simulink model "main_sim"  (Simulink 7.2)
settings: Solver=ode2  SolverMode=SingleTasking  StartTime=0.0  StopTime=tsim_max  FixedStep=dtsim  RelTol=1e-3
StopFcn:
  | %mkplt
undefined symbols (not defined in the file): aero_surf_qbar_off, aero_surf_qbar_on, assertion_time, att_type, att_type_numbers, bb_ellipsoid, bb_params, compute_all_rate_cols, compute_all_vel_cols, constants, cosA, DiscIntNeverNeededParam, dtsim, E_rwy, eow_boundary, full_surf_llim, full_surf_ulim, gain_set, gain_var_struct, MACH, MACH_att_fb, MACH_gain_mat, MACH_mass_IC, MACH_pos_IC, MACH_pqr_Bmat_IC, MACH_pqr_IC, MACH_pqr_u_IC, MACH_quat_IC, MACH_throttle_IC, MACH_U_nom_IC, MACH_vel_Bmat_IC, MACH_vel_cvdnom_IC, MACH_vel_IC, MACH_vel_uold_IC, max_LOS_rate, modes, N_rwy, pos, rcs_cvddes_thresh, reset_camcmd_on_entry, sinA, target_pos_IC, target_range_blind, target_range_detect, target_range_homing, target_vel_IC, trac_params, u_llim, u_ulim, use_auto_att_type, use_eow_as_iv, use_nav, use_pos_fltpath_lim, use_throt_estimate, use_variable_mass, use_wind_est, vel, vel_cmd_ramp_time, x_trac_IC
libraries: simulink x32, mach_lib x26, utility_lib x24, model_lib x15, simulink_need_slupdate x8, models x6
(part 3 of 5)

== system main_sim/claw_main/vel_loops/config_di ==
  cvd_nom : Inport  OutDataType=sfix(16)  OutScaling=2^0
  Bmat : Inport  Port=2  OutDataType=sfix(16)  OutScaling=2^0
  d_old : Inport  Port=3  OutDataType=sfix(16)  OutScaling=2^0
  d_nom : Inport  Port=4  OutDataType=sfix(16)  OutScaling=2^0
  cvd_des : Inport  Port=5  OutDataType=sfix(16)  OutScaling=2^0
  params : Inport  Port=6  OutDataType=sfix(16)  OutScaling=2^0
  di_smn : mach_lib/di_smn  SystemSampleTime=-1
  d_cmd : Outport  OutDataType=sfix(16)  OutScaling=2^0
  cvd_extra : Outport  Port=2  OutDataType=sfix(16)  OutScaling=2^0
  lambda : Outport  Port=3  OutDataType=sfix(16)  OutScaling=2^0
  solve_dat : Outport  Port=4  OutDataType=sfix(16)  OutScaling=2^0
  wires:
  cvd_nom/1 -> di_smn/1
  Bmat/1 -> di_smn/2
  d_old/1 -> di_smn/3
  d_nom/1 -> di_smn/4
  cvd_des/1 -> di_smn/5
  params/1 -> di_smn/6
  di_smn/1 -> d_cmd/1
  di_smn/2 -> cvd_extra/1
  di_smn/3 -> lambda/1
  di_smn/4 -> solve_dat/1

== system main_sim/claw_main/vel_loops/convert accel_cmd to NED_dd_cmd ==
  accel_cmd : Inport  OutDataType=sfix(16)  OutScaling=2^0
  accel_cmd_sw : Inport  Port=2  OutDataType=sfix(16)  OutScaling=2^0
  NEh_d : Inport  Port=3  OutDataType=sfix(16)  OutScaling=2^0
  Merge : Merge  InitialOutput=zeros(3,1)
  MinMax : MinMax  Function=max  OutDataType=sfix(16)  OutScaling=2^0
  NED_dd cmd : Subsystem  TreatAsAtomicUnit=on
  Switch Case : SwitchCase  CaseConditions={1,2}  CaseShowDefault=off
  vchigam_dot cmd : Subsystem  TreatAsAtomicUnit=on
  NEh_dd_cmd : Outport  OutDataType=sfix(16)  OutScaling=2^0
  wires:
  accel_cmd_sw/1 -> MinMax/1
  MinMax/1 -> Switch Case/1
  NEh_d/1 -> vchigam_dot cmd/2(NEh_d)
  vchigam_dot cmd/1(NEh_dd_cmd) -> Merge/2
  Merge/1 -> NEh_dd_cmd/1
  Switch Case/1 -> NED_dd cmd/Action
  Switch Case/2 -> vchigam_dot cmd/Action
  accel_cmd/1 -> vchigam_dot cmd/1(vchigam_dot_cmd), NED_dd cmd/1(NEH_dd_cmd_in)
  NED_dd cmd/1(NEh_dd_cmd) -> Merge/1

== system main_sim/claw_main/vel_loops/from inner ==
  att,T : Inport  OutDataType=sfix(16)  OutScaling=2^0
  Demux1 : Demux  Outputs=[ 2 1 MACH.num_u_throt ]
  Mux1 : Mux  Inputs=2
  Terminator : Terminator
  d_cmd : Outport  OutDataType=sfix(16)  OutScaling=2^0
  wires:
  att,T/1 -> Demux1/1
  Demux1/1 -> Mux1/1
  Mux1/1 -> d_cmd/1
  Demux1/3 -> Mux1/2
  Demux1/2 -> Terminator/1

== system main_sim/claw_main/vel_loops/from quat ==
  e,T : Inport  OutDataType=sfix(16)  OutScaling=2^0
  Demux1 : Demux  Outputs=[ 4 MACH.num_u_throt ]
  Mux1 : Mux  Inputs=2
  Selector1 : Selector  InputPortWidth=3  IndexOptions=Index vector (dialog)  Indices=1:2  OutputSizes=1
  e2att : utility_lib/e2att  SystemSampleTime=-1
  d_cmd : Outport  OutDataType=sfix(16)  OutScaling=2^0
  wires:
  e2att/1 -> Selector1/1
  Selector1/1 -> Mux1/1
  Demux1/2 -> Mux1/2
  Mux1/1 -> d_cmd/1
  Demux1/1 -> e2att/1
  e,T/1 -> Demux1/1

== system main_sim/claw_main/vel_loops/select vel cmd ==
  NEh_dot_current : Inport  OutDataType=sfix(16)  OutScaling=2^0
  cam_current : Inport  Port=2  OutDataType=sfix(16)  OutScaling=2^0
  outer cmd : Inport  Port=3  OutDataType=sfix(16)  OutScaling=2^0
  signal_bus : Inport  Port=4  OutDataType=sfix(16)  OutScaling=2^0
  Bus Selector : BusSelector  OutputSignals=cmd_bus.select_cmd.vel,cmd_bus.autopilot_cmd
  Demux3 : Demux  Outputs=[ MACH.vel_num_cv 1 ]
  Multiport Switch : MultiPortSwitch  zeroidx=on  SaturateOnIntegerOverflow=on
  Mux : Mux  Inputs=2
  Selector1 : Selector  InputPortWidth=4  IndexOptions=Index vector (dialog)  Indices=[1 2 4 3]  OutputSizes=1
  Selector2 : Selector  InputPortWidth=4  IndexOptions=Index vector (dialog)  Indices=[1 2 4 3]  OutputSizes=1
  NEh_dot_cmd : Outport  OutDataType=sfix(16)  OutScaling=2^0
  cam_cmd : Outport  Port=2  OutDataType=sfix(16)  OutScaling=2^0
  cmd : Outport  Port=3  OutDataType=sfix(16)  OutScaling=2^0
  wires:
  Multiport Switch/1 -> cmd/1, Selector2/1
  outer cmd/1 -> Multiport Switch/4
  Bus Selector/1 -> Multiport Switch/1  "<vel>"
  Selector2/1 -> Demux3/1
  Demux3/1 -> NEh_dot_cmd/1
  Demux3/2 -> cam_cmd/1
  Mux/1 -> Selector1/1
  NEh_dot_current/1 -> Mux/1
  Selector1/1 -> Multiport Switch/2
  signal_bus/1 -> Bus Selector/1
  Bus Selector/2 -> Multiport Switch/3  "<autopilot_cmd>"
  cam_current/1 -> Mux/2

== system main_sim/claw_main/vel_loops/set di params ==
  note: Note: dc_fltpath is now computed from NEh_dot.
      | Switch to recover old computation base on NEh_dot_cmd
  NEh_dot_cmd : Inport  OutDataType=sfix(16)  OutScaling=2^0
  full_surf : Inport  Port=2  OutDataType=sfix(16)  OutScaling=2^0
  u_old : Inport  Port=3  OutDataType=sfix(16)  OutScaling=2^0
  uvw : Inport  Port=4  OutDataType=sfix(16)  OutScaling=2^0
  dc_fltpath : Inport  Port=5  OutDataType=sfix(16)  OutScaling=2^0
  Bus Creator1 : BusCreator  Inputs=7
  Bus Selector : BusSelector  OutputSignals=u_ulim,u_llim,u_urlim,u_lrlim
  Bus Selector1 : BusSelector  OutputSignals=throt_ulim,throt_llim
  Constant1 : Constant  Value=MACH.vel_wght_cv  OutDataType=sfix(16)  OutScaling=2^0
  Constant3 : Constant  Value=MACH.vel_u_pref  OutDataType=sfix(16)  OutScaling=2^0
  Constant4 : Constant  Value=MACH.vel_wght_u_pref  OutDataType=sfix(16)  OutScaling=2^0
  Demux1 : Demux  Outputs=[ 2 MACH.num_u_throt ]
  Gain2 : Gain  Gain=repmat(MACH.vel_wght_fltpath',1,3)  ParameterDataType=sfix(16)  ParameterScaling=2^0  OutDataType=sfix(16)  OutScaling=2^0
  Logical Operator : Logic  Inputs=1  AllPortsSameDT=off  OutDataTypeMode=boolean  OutDataTypeStr=boolean
  Manual Switch : simulink/Signal Routing/Manual Switch  SystemSampleTime=-1  sw=1  action=0  varsize=off
  Multiport Switch2 : MultiPortSwitch  Inputs=2  zeroidx=on
  Relational Operator : RelationalOperator  Operator===  LogicOutDataTypeMode=boolean  OutDataTypeStr=boolean
  Terminator : Terminator
  att limits : Subsystem
  combine limits : Subsystem
  compute dc_fltpath : Subsystem
  throttle limits : Subsystem
  params : Outport  OutDataType=sfix(16)  OutScaling=2^0
  wires:
  Constant4/1 -> Bus Creator1/6  "wght_u_pref"
  Constant3/1 -> Bus Creator1/5  "u_pref"
  Multiport Switch2/1 -> Bus Creator1/7  "wght_cv"
  Constant1/1 -> Multiport Switch2/2
  full_surf/1 -> throttle limits/1(full_surf)
  Bus Selector/1 -> Bus Creator1/1  "<u_ulim>"
  Bus Selector/2 -> Bus Creator1/2  "<u_llim>"
  Bus Selector/4 -> Bus Creator1/4  "<u_lrlim>"
  Bus Creator1/1 -> params/1
  Relational Operator/1 -> Logical Operator/1
  Logical Operator/1 -> Multiport Switch2/1
  uvw/1 -> att limits/1(uvw)
  att limits/1(att_limits) -> combine limits/1(att_limits)
  throttle limits/1(throt_limits) -> combine limits/2(throt_limits), Bus Selector1/1
  combine limits/1(vel_u_limits) -> Bus Selector/1
  Bus Selector/3 -> Bus Creator1/3  "<u_urlim>"
  Bus Selector1/1 -> Relational Operator/1  "<throt_ulim>"
  Bus Selector1/2 -> Relational Operator/2  "<throt_llim>"
  Demux1/2 -> throttle limits/2(throt_old)
  Demux1/1 -> Terminator/1
  u_old/1 -> Demux1/1
  Gain2/1 -> Multiport Switch2/3
  NEh_dot_cmd/1 -> compute dc_fltpath/1(NEh_dot_fltpath)
  Manual Switch/1 -> Gain2/1
  dc_fltpath/1 -> Manual Switch/1
  compute dc_fltpath/1(dc_fltpath) -> Manual Switch/2

== system main_sim/claw_main/vel_loops/to full att/e cmd ==
  d_cmd : Inport  OutDataType=sfix(16)  OutScaling=2^0
  cam : Inport  Port=2  OutDataType=sfix(16)  OutScaling=2^0
  Demux : Demux  Outputs=[ 2 MACH.num_u_throt ]
  Mux : Mux  Inputs=2
  Mux1 : Mux  Inputs=2
  Mux4 : Mux  Inputs=2
  att2e : utility_lib/att2e  SystemSampleTime=-1  quat_IC=MACH_quat_IC
  att,T : Outport  OutDataType=sfix(16)  OutScaling=2^0
  e,T : Outport  Port=2  OutDataType=sfix(16)  OutScaling=2^0
  wires:
  Demux/2 -> Mux/2, Mux1/2  "throt"
  Demux/1 -> Mux4/1
  cam/1 -> Mux4/2
  Mux4/1 -> Mux/1, att2e/1  "att"
  d_cmd/1 -> Demux/1
  Mux/1 -> att,T/1
  att2e/1 -> Mux1/1
  Mux1/1 -> e,T/1

== system main_sim/claw_main/vel_loops/xu2d ==
  X : Inport  OutDataType=sfix(16)  OutScaling=2^0
  U : Inport  Port=2  OutDataType=sfix(16)  OutScaling=2^0
  params : Inport  Port=3  OutDataType=sfix(16)  OutScaling=2^0
  Assignment : Assignment  IndexOptions=Index vector (dialog)  Indices=MACH.throttle_idx  OutputSizes=[1 1]
  Bus Selector : BusSelector  OutputSignals=u_llim,u_ulim
  Demux : Demux  Outputs=[ 2 1 ]
  MinMax : MinMax  Inputs=2  OutDataType=sfix(16)  OutScaling=2^0  SaturateOnIntegerOverflow=on  InputSameDT=on
  MinMax1 : MinMax  Function=max  Inputs=2  OutDataType=sfix(16)  OutScaling=2^0  SaturateOnIntegerOverflow=on  InputSameDT=on
  Mux : Mux  Inputs=2
  Reshape : Reshape
  Selector1 : Selector  InputPortWidth=MACH.num_x  IndexOptions=Index vector (dialog)  Indices=MACH.quat_idx  OutputSizes=1
  Selector2 : Selector  InputPortWidth=MACH.num_u  IndexOptions=Index vector (dialog)  Indices=MACH.throttle_idx  OutputSizes=1
  Selector3 : Selector  InputPortWidth=MACH.vel_num_u  IndexOptions=Index vector (dialog)  Indices=3:MACH.vel_num_u  OutputSizes=1
  Selector4 : Selector  InputPortWidth=MACH.vel_num_u  IndexOptions=Index vector (dialog)  Indices=3:MACH.vel_num_u  OutputSizes=1
  e2att : utility_lib/e2att  SystemSampleTime=-1
  U_limited : Outport  OutDataType=sfix(16)  OutScaling=2^0
  d_nom : Outport  Port=2  OutDataType=sfix(16)  OutScaling=2^0
  cam : Outport  Port=3  OutDataType=sfix(16)  OutScaling=2^0
  wires:
  Selector1/1 -> e2att/1
  Selector2/1 -> MinMax1/1  "throttle"
  Mux/1 -> d_nom/1
  X/1 -> Selector1/1
  U/1 -> Selector2/1, Assignment/1
  Demux/1 -> Mux/1
  Demux/2 -> cam/1
  params/1 -> Bus Selector/1
  Bus Selector/1 -> Selector3/1  "<u_llim>"
  MinMax1/1 -> MinMax/1
  Bus Selector/2 -> Selector4/1  "<u_ulim>"
  Selector4/1 -> MinMax/2
  Selector3/1 -> MinMax1/2
  MinMax/1 -> Assignment/2, Reshape/1
  Assignment/1 -> U_limited/1
  e2att/1 -> Demux/1
  Reshape/1 -> Mux/2

== system main_sim/vehicle_model/target/seeker model/seeker model ==
  NEh_target : Inport  OutDataType=sfix(16)  OutScaling=2^0
  NEh_d_target : Inport  Port=2  OutDataType=sfix(16)  OutScaling=2^0
  NEh : Inport  Port=3  OutDataType=sfix(16)  OutScaling=2^0
  NEh_d : Inport  Port=4  OutDataType=sfix(16)  OutScaling=2^0
  Bus Creator : BusCreator  Inputs=2
  Product1 : Product  Multiplication=Matrix(*)  OutDataType=sfix(16)  OutScaling=2^0  RndMeth=Zero
  Reshape : Reshape  OutputDimensionality=Customize  OutputDimensions=[3 3]
  Selector : Selector  NumberOfDimensions=2  InputPortWidth=3  IndexOptions=Index vector (dialog),Select all  Indices=2:3,-1  OutputSizes=1
  Sum : Sum  Inputs=|+-  OutDataType=sfix(16)  OutScaling=2^0
  Sum1 : Sum  Inputs=|+-  OutDataType=sfix(16)  OutScaling=2^0
  cart to polar : Subsystem
  convert to NED : Gain  Gain=[1 1 -1]  ParameterDataType=sfix(16)  ParameterScaling=2^0  OutDataType=sfix(16)  OutScaling=2^0
  convert to NED_d : Gain  Gain=[1 1 -1]  ParameterDataType=sfix(16)  ParameterScaling=2^0  OutDataType=sfix(16)  OutScaling=2^0
  vec2dc : utility_lib/vec2dc  SystemSampleTime=-1
  seeker : Outport  OutDataType=sfix(16)  OutScaling=2^0
  wires:
  cart to polar/1(LOS_rate) -> Bus Creator/1  "LOS_rate"
  NEh_d_target/1 -> Sum1/1
  NEh_target/1 -> Sum/1
  NEh_d/1 -> Sum1/2
  NEh/1 -> Sum/2
  convert to NED_d/1 -> Product1/2
  Product1/1 -> cart to polar/2(cross_d;vert_d)
  Sum1/1 -> convert to NED_d/1
  Selector/1 -> Product1/1
  convert to NED/1 -> vec2dc/1
  Sum/1 -> convert to NED/1
  Reshape/1 -> Selector/1
  vec2dc/1 -> Reshape/1
  vec2dc/2 -> cart to polar/1(scaling info), Bus Creator/2  "aux_info"
  Bus Creator/1 -> seeker/1

== system main_sim/claw_main/att_loops/dyn inv/Limit rate cmd ==
  limit_pqr_cmd : Inport  OutDataType=sfix(16)  OutScaling=2^0
  uvw : Inport  Port=2  OutDataType=sfix(16)  OutScaling=2^0
  pqr : Inport  Port=3  OutDataType=sfix(16)  OutScaling=2^0
  Constant1 : Constant  Value=MACH.az_llim  OutDataType=sfix(16)  OutScaling=2^0
  Constant2 : Constant  Value=MACH.att_u_llim  OutDataType=sfix(16)  OutScaling=2^0
  Constant3 : Constant  Value=MACH.att_u_ulim  OutDataType=sfix(16)  OutScaling=2^0
  Constant4 : Constant  Value=MACH.az_ulim  OutDataType=sfix(16)  OutScaling=2^0
  Enforce lower limit : MinMax  Function=max  Inputs=2  OutDataType=sfix(16)  OutScaling=2^-10  OutDataTypeStr=Inherit: Inherit via back propagation  ZeroCross=off
  Enforce upper limit : MinMax  Inputs=2  OutDataType=sfix(16)  OutScaling=2^-10  OutDataTypeStr=Inherit: Inherit via back propagation  ZeroCross=off
  Multiport Switch : MultiPortSwitch  Inputs=2  zeroidx=on
  velocity based angular rate llim : mach_lib/velocity based angular rate limit  SystemSampleTime=-1  q_idx=2
  velocity based angular rate ulim : mach_lib/velocity based angular rate limit  SystemSampleTime=-1  q_idx=2
  pqr_limited : Outport  OutDataType=sfix(16)  OutScaling=2^0
  wires:
  Enforce lower limit/1 -> Enforce upper limit/1
  pqr/1 -> Enforce lower limit/1, Multiport Switch/2
  velocity based angular rate ulim/1 -> Enforce upper limit/2
  uvw/1 -> velocity based angular rate ulim/3, velocity based angular rate llim/3
  Constant2/1 -> velocity based angular rate llim/1
  Constant4/1 -> velocity based angular rate llim/2
  Constant1/1 -> velocity based angular rate ulim/2
  Constant3/1 -> velocity based angular rate ulim/1  "upper_limit"
  velocity based angular rate llim/1 -> Enforce lower limit/2
  Enforce upper limit/1 -> Multiport Switch/3
  Multiport Switch/1 -> pqr_limited/1
  limit_pqr_cmd/1 -> Multiport Switch/1

== system main_sim/claw_main/att_loops/select att cmd/get direct cmd ==
  signal_bus : Inport  OutDataType=sfix(16)  OutScaling=2^0
  Bus Selector : BusSelector  OutputSignals=cmd_bus.autopilot_cmd,mode_sw.full_surf_cmd_sw,full_surf.full_surf_cmd
  Demux1 : Demux  Outputs=[ 3 1 ]
  Gain : Gain  Gain=MACH.throt_mixer  ParameterDataType=sfix(16)  ParameterScaling=2^0  OutDataType=sfix(16)  OutScaling=2^0
  Multiport Switch2 : MultiPortSwitch  Inputs=2  zeroidx=on
  throttle : Selector  InputPortWidth=MACH.num_u  IndexOptions=Index vector (dialog)  Indices=MACH.throttle_idx  OutputSizes=1
  att : Outport  OutDataType=sfix(16)  OutScaling=2^0
  throt : Outport  Port=2  OutDataType=sfix(16)  OutScaling=2^0
  wires:
  Demux1/1 -> att/1
  Demux1/2 -> Gain/1
  signal_bus/1 -> Bus Selector/1
  Bus Selector/1 -> Demux1/1  "<autopilot_cmd>"
  Bus Selector/2 -> Multiport Switch2/1  "<full_surf_cmd_sw>"
  Gain/1 -> Multiport Switch2/2
  Bus Selector/3 -> throttle/1  "<full_surf_cmd>"
  throttle/1 -> Multiport Switch2/3
  Multiport Switch2/1 -> throt/1

== system main_sim/claw_main/grab ExportedGlobal/grab cv variables/Subsystem ==
  In1 : Inport  OutDataType=sfix(16)  OutScaling=2^0
  In2 : Inport  Port=2  OutDataType=sfix(16)  OutScaling=2^0
  In3 : Inport  Port=3  OutDataType=sfix(16)  OutScaling=2^0
  In4 : Inport  Port=4  OutDataType=sfix(16)  OutScaling=2^0
  In5 : Inport  Port=5  OutDataType=sfix(16)  OutScaling=2^0
  In6 : Inport  Port=6  OutDataType=sfix(16)  OutScaling=2^0
  In7 : Inport  Port=7  OutDataType=sfix(16)  OutScaling=2^0
  In8 : Inport  Port=8  OutDataType=sfix(16)  OutScaling=2^0
  In9 : Inport  Port=9  OutDataType=sfix(16)  OutScaling=2^0
  In10 : Inport  Port=10  OutDataType=sfix(16)  OutScaling=2^0
  In11 : Inport  Port=11  OutDataType=sfix(16)  OutScaling=2^0
  In12 : Inport  Port=12  OutDataType=sfix(16)  OutScaling=2^0
  In13 : Inport  Port=13  OutDataType=sfix(16)  OutScaling=2^0
  Out1 : Outport  OutDataType=sfix(16)  OutScaling=2^0
  Out2 : Outport  Port=2  OutDataType=sfix(16)  OutScaling=2^0
  Out3 : Outport  Port=3  OutDataType=sfix(16)  OutScaling=2^0
  Out4 : Outport  Port=4  OutDataType=sfix(16)  OutScaling=2^0
  Out5 : Outport  Port=5  OutDataType=sfix(16)  OutScaling=2^0
  Out6 : Outport  Port=6  OutDataType=sfix(16)  OutScaling=2^0
  Out7 : Outport  Port=7  OutDataType=sfix(16)  OutScaling=2^0
  Out8 : Outport  Port=8  OutDataType=sfix(16)  OutScaling=2^0
  Out9 : Outport  Port=9  OutDataType=sfix(16)  OutScaling=2^0
  Out10 : Outport  Port=10  OutDataType=sfix(16)  OutScaling=2^0
  Out11 : Outport  Port=11  OutDataType=sfix(16)  OutScaling=2^0
  Out12 : Outport  Port=12  OutDataType=sfix(16)  OutScaling=2^0
  Out13 : Outport  Port=13  OutDataType=sfix(16)  OutScaling=2^0
  wires:
  In1/1 -> Out1/1
  In2/1 -> Out2/1
  In3/1 -> Out3/1
  In4/1 -> Out4/1
  In5/1 -> Out5/1
  In6/1 -> Out6/1
  In7/1 -> Out7/1
  In8/1 -> Out8/1
  In9/1 -> Out9/1
  In10/1 -> Out10/1
  In11/1 -> Out11/1
  In12/1 -> Out12/1
  In13/1 -> Out13/1

== system main_sim/claw_main/grab ExportedGlobal/grab cvcmd variables/Subsystem ==
  In1 : Inport  OutDataType=sfix(16)  OutScaling=2^0
  In2 : Inport  Port=2  OutDataType=sfix(16)  OutScaling=2^0
  In3 : Inport  Port=3  OutDataType=sfix(16)  OutScaling=2^0
  In4 : Inport  Port=4  OutDataType=sfix(16)  OutScaling=2^0
  In5 : Inport  Port=5  OutDataType=sfix(16)  OutScaling=2^0
  In6 : Inport  Port=6  OutDataType=sfix(16)  OutScaling=2^0
  In7 : Inport  Port=7  OutDataType=sfix(16)  OutScaling=2^0
  In8 : Inport  Port=8  OutDataType=sfix(16)  OutScaling=2^0
  In9 : Inport  Port=9  OutDataType=sfix(16)  OutScaling=2^0
  In10 : Inport  Port=10  OutDataType=sfix(16)  OutScaling=2^0
  In11 : Inport  Port=11  OutDataType=sfix(16)  OutScaling=2^0
  In12 : Inport  Port=12  OutDataType=sfix(16)  OutScaling=2^0
  In13 : Inport  Port=13  OutDataType=sfix(16)  OutScaling=2^0
  Out1 : Outport  OutDataType=sfix(16)  OutScaling=2^0
  Out2 : Outport  Port=2  OutDataType=sfix(16)  OutScaling=2^0
  Out3 : Outport  Port=3  OutDataType=sfix(16)  OutScaling=2^0
  Out4 : Outport  Port=4  OutDataType=sfix(16)  OutScaling=2^0
  Out5 : Outport  Port=5  OutDataType=sfix(16)  OutScaling=2^0
  Out6 : Outport  Port=6  OutDataType=sfix(16)  OutScaling=2^0
  Out7 : Outport  Port=7  OutDataType=sfix(16)  OutScaling=2^0
  Out8 : Outport  Port=8  OutDataType=sfix(16)  OutScaling=2^0
  Out9 : Outport  Port=9  OutDataType=sfix(16)  OutScaling=2^0
  Out10 : Outport  Port=10  OutDataType=sfix(16)  OutScaling=2^0
  Out11 : Outport  Port=11  OutDataType=sfix(16)  OutScaling=2^0
  Out12 : Outport  Port=12  OutDataType=sfix(16)  OutScaling=2^0
  Out13 : Outport  Port=13  OutDataType=sfix(16)  OutScaling=2^0
  wires:
  In1/1 -> Out1/1
  In2/1 -> Out2/1
  In3/1 -> Out3/1
  In4/1 -> Out4/1
  In5/1 -> Out5/1
  In6/1 -> Out6/1
  In7/1 -> Out7/1
  In8/1 -> Out8/1
  In9/1 -> Out9/1
  In10/1 -> Out10/1
  In11/1 -> Out11/1
  In12/1 -> Out12/1
  In13/1 -> Out13/1

== system main_sim/claw_main/grab ExportedGlobal/grab cvdex variables/Subsystem ==
  In1 : Inport  OutDataType=sfix(16)  OutScaling=2^0
  In2 : Inport  Port=2  OutDataType=sfix(16)  OutScaling=2^0
  In3 : Inport  Port=3  OutDataType=sfix(16)  OutScaling=2^0
  In4 : Inport  Port=4  OutDataType=sfix(16)  OutScaling=2^0
  In5 : Inport  Port=5  OutDataType=sfix(16)  OutScaling=2^0
  In6 : Inport  Port=6  OutDataType=sfix(16)  OutScaling=2^0
  In7 : Inport  Port=7  OutDataType=sfix(16)  OutScaling=2^0
  In8 : Inport  Port=8  OutDataType=sfix(16)  OutScaling=2^0
  In9 : Inport  Port=9  OutDataType=sfix(16)  OutScaling=2^0
  In10 : Inport  Port=10  OutDataType=sfix(16)  OutScaling=2^0
  In11 : Inport  Port=11  OutDataType=sfix(16)  OutScaling=2^0
  In12 : Inport  Port=12  OutDataType=sfix(16)  OutScaling=2^0
  In13 : Inport  Port=13  OutDataType=sfix(16)  OutScaling=2^0
  Out1 : Outport  OutDataType=sfix(16)  OutScaling=2^0
  Out2 : Outport  Port=2  OutDataType=sfix(16)  OutScaling=2^0
  Out3 : Outport  Port=3  OutDataType=sfix(16)  OutScaling=2^0
  Out4 : Outport  Port=4  OutDataType=sfix(16)  OutScaling=2^0
  Out5 : Outport  Port=5  OutDataType=sfix(16)  OutScaling=2^0
  Out6 : Outport  Port=6  OutDataType=sfix(16)  OutScaling=2^0
  Out7 : Outport  Port=7  OutDataType=sfix(16)  OutScaling=2^0
  Out8 : Outport  Port=8  OutDataType=sfix(16)  OutScaling=2^0
  Out9 : Outport  Port=9  OutDataType=sfix(16)  OutScaling=2^0
  Out10 : Outport  Port=10  OutDataType=sfix(16)  OutScaling=2^0
  Out11 : Outport  Port=11  OutDataType=sfix(16)  OutScaling=2^0
  Out12 : Outport  Port=12  OutDataType=sfix(16)  OutScaling=2^0
  Out13 : Outport  Port=13  OutDataType=sfix(16)  OutScaling=2^0
  wires:
  In1/1 -> Out1/1
  In2/1 -> Out2/1
  In3/1 -> Out3/1
  In4/1 -> Out4/1
  In5/1 -> Out5/1
  In6/1 -> Out6/1
  In7/1 -> Out7/1
  In8/1 -> Out8/1
  In9/1 -> Out9/1
  In10/1 -> Out10/1
  In11/1 -> Out11/1
  In12/1 -> Out12/1
  In13/1 -> Out13/1

== system main_sim/claw_main/grab ExportedGlobal/grab integrator variables/Subsystem ==
  In1 : Inport  OutDataType=sfix(16)  OutScaling=2^0
  In2 : Inport  Port=2  OutDataType=sfix(16)  OutScaling=2^0
  In3 : Inport  Port=3  OutDataType=sfix(16)  OutScaling=2^0
  In4 : Inport  Port=4  OutDataType=sfix(16)  OutScaling=2^0
  In5 : Inport  Port=5  OutDataType=sfix(16)  OutScaling=2^0
  In6 : Inport  Port=6  OutDataType=sfix(16)  OutScaling=2^0
  In7 : Inport  Port=7  OutDataType=sfix(16)  OutScaling=2^0
  In8 : Inport  Port=8  OutDataType=sfix(16)  OutScaling=2^0
  In9 : Inport  Port=9  OutDataType=sfix(16)  OutScaling=2^0
  In10 : Inport  Port=10  OutDataType=sfix(16)  OutScaling=2^0
  In11 : Inport  Port=11  OutDataType=sfix(16)  OutScaling=2^0
  In12 : Inport  Port=12  OutDataType=sfix(16)  OutScaling=2^0
  In13 : Inport  Port=13  OutDataType=sfix(16)  OutScaling=2^0
  Out1 : Outport  OutDataType=sfix(16)  OutScaling=2^0
  Out2 : Outport  Port=2  OutDataType=sfix(16)  OutScaling=2^0
  Out3 : Outport  Port=3  OutDataType=sfix(16)  OutScaling=2^0
  Out4 : Outport  Port=4  OutDataType=sfix(16)  OutScaling=2^0
  Out5 : Outport  Port=5  OutDataType=sfix(16)  OutScaling=2^0
  Out6 : Outport  Port=6  OutDataType=sfix(16)  OutScaling=2^0
  Out7 : Outport  Port=7  OutDataType=sfix(16)  OutScaling=2^0
  Out8 : Outport  Port=8  OutDataType=sfix(16)  OutScaling=2^0
  Out9 : Outport  Port=9  OutDataType=sfix(16)  OutScaling=2^0
  Out10 : Outport  Port=10  OutDataType=sfix(16)  OutScaling=2^0
  Out11 : Outport  Port=11  OutDataType=sfix(16)  OutScaling=2^0
  Out12 : Outport  Port=12  OutDataType=sfix(16)  OutScaling=2^0
  Out13 : Outport  Port=13  OutDataType=sfix(16)  OutScaling=2^0
  wires:
  In1/1 -> Out1/1
  In2/1 -> Out2/1
  In3/1 -> Out3/1
  In4/1 -> Out4/1
  In5/1 -> Out5/1
  In6/1 -> Out6/1
  In7/1 -> Out7/1
  In8/1 -> Out8/1
  In9/1 -> Out9/1
  In10/1 -> Out10/1
  In11/1 -> Out11/1
  In12/1 -> Out12/1
  In13/1 -> Out13/1

== system main_sim/claw_main/grab ExportedGlobal/grab w_est variables/Subsystem ==
  In1 : Inport  OutDataType=sfix(16)  OutScaling=2^0
  In2 : Inport  Port=2  OutDataType=sfix(16)  OutScaling=2^0
  In3 : Inport  Port=3  OutDataType=sfix(16)  OutScaling=2^0
  Out1 : Outport  OutDataType=sfix(16)  OutScaling=2^0
  Out2 : Outport  Port=2  OutDataType=sfix(16)  OutScaling=2^0
  Out3 : Outport  Port=3  OutDataType=sfix(16)  OutScaling=2^0
  wires:
  In1/1 -> Out1/1
  In2/1 -> Out2/1
  In3/1 -> Out3/1

== system main_sim/claw_main/input processing/mode dependent stick processing/att rate cmd ==
  note: In attitude, velocity, position mode, while enabled,
      | replace cam command with integrated rate command.
      |
      | In attitude mode, while enabled,
      | replace the other att commands with integrated rate commands.
      |
      | integrators are set to current values upon transition into this condition.
      | Reset of cam cmd can be disabled by setting
      | reset_camcmd_on_entry to false.
      |
      | In addition to specified conditions, reset also occurs, if applicable
      | when att_type changes
  mode : Inport  OutDataType=sfix(16)  OutScaling=2^0
  command_in : Inport  Port=2  OutDataType=sfix(16)  OutScaling=2^0
  signal_bus : Inport  Port=3  OutDataType=sfix(16)  OutScaling=2^0
  Bus Selector3 : BusSelector  OutputSignals=mode_sw.att_rate_cmd_sw,mode_sw.cam_rate_cmd_sw,y_meas.dircos
  Compare To Constant1 : simulink/Logic and Bit Operations/Compare To Constant  SystemSampleTime=-1  relop===  const=modes.att  LogicOutDataTypeMode=boolean  ZeroCross=off
  Compare To Constant2 : simulink/Logic and Bit Operations/Compare To Constant  SystemSampleTime=-1  relop=>=  const=modes.att  LogicOutDataTypeMode=boolean  ZeroCross=off
  Gain1 : Gain  Gain=[ 1 1 reset_camcmd_on_entry ]  ParameterDataType=sfix(16)  ParameterScaling=2^0  OutDataType=sfix(16)  OutScaling=2^0
  Logical Operator1 : Logic  Operator=OR  AllPortsSameDT=off
  Logical Operator2 : Logic  AllPortsSameDT=off
  Logical Operator4 : Logic  AllPortsSameDT=off
  Multiport Switch1 : MultiPortSwitch  Inputs=2  zeroidx=on
  Mux : Mux  Inputs=3
  Product1 : Product  OutDataType=sfix(16)  OutScaling=2^0  RndMeth=Zero
  also reset att on att_type change : Subsystem
  att cmd integration : DiscreteIntegrator  ExternalReset=either  InitialConditionSource=external  SampleTime=-1  OutDataType=sfix(16)  OutScaling=2^0  ICPrevOutput=DiscIntNeverNeededParam  ICPrevScaledInput=DiscIntNeverNeededParam
  att/att rate cmd : Selector  InputPortWidth=4  IndexOptions=Index vector (dialog)  Indices=1:3  OutputSizes=1
  dc2att : utility_lib/dc2att  SystemSampleTime=-1
  set att cmd : Assignment  IndexOptions=Index vector (dialog)  Indices=1:3  OutputSizes=[1 1]
  command_out : Outport  OutDataType=sfix(16)  OutScaling=2^0
  wires:
  Product1/1 -> att cmd integration/1
  Gain1/1 -> att cmd integration/2
  att cmd integration/1 -> Multiport Switch1/3
  also reset att on att_type change/1(reset_out) -> Gain1/1
  mode/1 -> Compare To Constant1/1, Compare To Constant2/1
  command_in/1 -> set att cmd/1, att/att rate cmd/1
  Compare To Constant1/1 -> Logical Operator4/1
  att/att rate cmd/1 -> Product1/1, Multiport Switch1/2
  Logical Operator4/1 -> Mux/1, Mux/2
  Logical Operator1/1 -> Logical Operator2/1
  Logical Operator2/1 -> Mux/3
  Compare To Constant2/1 -> Logical Operator2/2
  Mux/1 -> Product1/2, also reset att on att_type change/1(reset_in), Multiport Switch1/1
  Multiport Switch1/1 -> set att cmd/2
  set att cmd/1 -> command_out/1
  dc2att/1 -> att cmd integration/3
  signal_bus/1 -> Bus Selector3/1
  Bus Selector3/1 -> Logical Operator4/2, Logical Operator1/1  "<att_rate_cmd_sw>"
  Bus Selector3/2 -> Logical Operator1/2  "<cam_rate_cmd_sw>"
  Bus Selector3/3 -> dc2att/1  "<dircos>"

== system main_sim/claw_main/input processing/mode dependent stick processing/att_type cmd ==
  mode : Inport  OutDataType=sfix(16)  OutScaling=2^0
  command_in : Inport  Port=2  OutDataType=sfix(16)  OutScaling=2^0
  signal_bus : Inport  Port=3  OutDataType=sfix(16)  OutScaling=2^0
  Bus Selector3 : BusSelector  OutputSignals=mode_sw.att_type
  Compare To Constant1 : simulink/Logic and Bit Operations/Compare To Constant  SystemSampleTime=-1  relop===  const=modes.att  LogicOutDataTypeMode=boolean  ZeroCross=off
  Constant4 : Constant  Value=use_auto_att_type  OutDataType=sfix(16)  OutScaling=2^0
  From Workspace1 : FromWorkspace  VariableName=rpy_cmd_fw  SampleTime=MACH.dt  OutputAfterFinalValue=Holding final value
  From Workspace2 : FromWorkspace  VariableName=mab_cmd_fw  SampleTime=MACH.dt  OutputAfterFinalValue=Holding final value
  From Workspace4 : FromWorkspace  VariableName=tiltcam_cmd_fw  SampleTime=MACH.dt  OutputAfterFinalValue=Holding final value
  Logical Operator4 : Logic  AllPortsSameDT=off
  Multiport Switch1 : MultiPortSwitch  Inputs=2  zeroidx=on
  Multiport Switch2 : MultiPortSwitch  Inputs=length(att_type_numbers)
  att cmd : Selector  InputPortWidth=4  IndexOptions=Index vector (dialog)  Indices=1:3  OutputSizes=1
  bam_cmd : Selector  InputPortWidth=3  IndexOptions=Index vector (dialog)  Indices=[3 2 1]  OutputSizes=1
  set att cmd : Assignment  IndexOptions=Index vector (dialog)  Indices=1:3  OutputSizes=[1 1]
  ypr_cmd : Selector  InputPortWidth=3  IndexOptions=Index vector (dialog)  Indices=[3 2 1]  OutputSizes=1
  command_out : Outport  OutDataType=sfix(16)  OutScaling=2^0
  wires:
  signal_bus/1 -> Bus Selector3/1
  set att cmd/1 -> command_out/1
  Multiport Switch1/1 -> set att cmd/2
  Logical Operator4/1 -> Multiport Switch1/1
  att cmd/1 -> Multiport Switch1/2
  Compare To Constant1/1 -> Logical Operator4/1
  command_in/1 -> att cmd/1, set att cmd/1
  mode/1 -> Compare To Constant1/1
  Constant4/1 -> Logical Operator4/2
  Bus Selector3/1 -> Multiport Switch2/1  "<att_type>"
  From Workspace4/1 -> Multiport Switch2/2
  From Workspace2/1 -> Multiport Switch2/5, bam_cmd/1
  From Workspace1/1 -> Multiport Switch2/3, ypr_cmd/1
  bam_cmd/1 -> Multiport Switch2/6
  Multiport Switch2/1 -> Multiport Switch1/3
  ypr_cmd/1 -> Multiport Switch2/4

== system main_sim/claw_main/input processing/mode dependent stick processing/feed forward ==
  table_bus : Inport  OutDataType=sfix(16)  OutScaling=2^0
  signal_bus : Inport  Port=2  OutDataType=sfix(16)  OutScaling=2^0
  Bus Creator : BusCreator
  Bus Selector : BusSelector  OutputSignals=eow_idx,eow_large,X_idx
  Constant : Constant  Value=use_eow_as_iv  OutDataType=sfix(16)  OutScaling=2^0
  Constant1 : Constant  Value=zeros(MACH.pqr_num_cv,1)  OutDataType=sfix(16)  OutScaling=2^0
  From Workspace1 : FromWorkspace  VariableName=vel_ff_fw  SampleTime=MACH.dt  OutputAfterFinalValue=Holding final value
  From Workspace4 : FromWorkspace  VariableName=pos_ff_fw  SampleTime=MACH.dt  OutputAfterFinalValue=Holding final value
  Switch{,1..3} (4 alike) : Switch  Threshold=0.5
  get att_ff : Subsystem
  lookup using  energy over weight : Subsystem
  "lookup using X  " : Subsystem
  feed_forward : Outport  OutDataType=sfix(16)  OutScaling=2^0
  wires:
  Switch/1 -> Bus Creator/1  "pos_ff"
  Switch1/1 -> Bus Creator/2  "vel_ff"
  get att_ff/1(att_ff) -> Bus Creator/3  "att_ff"
  Constant1/1 -> Bus Creator/4  "pqr_ff"
  Bus Creator/1 -> feed_forward/1
  From Workspace4/1 -> Switch/3
  From Workspace1/1 -> Switch1/3
  Constant/1 -> Switch1/2, Switch/2
  Switch2/1 -> Switch/1
  lookup using  energy over weight/1(pos_ff) -> Switch2/1
  Switch3/1 -> Switch1/1
  lookup using  energy over weight/2(vel_ff) -> Switch3/1
  "lookup using X  "/2(vel_ff) -> Switch3/3
  "lookup using X  "/1(pos_ff) -> Switch2/3
  table_bus/1 -> Bus Selector/1
  Bus Selector/1 -> lookup using  energy over weight/1(eow_idx)  "<eow_idx>"
  Bus Selector/2 -> Switch2/2, Switch3/2  "<eow_large>"
  Bus Selector/3 -> "lookup using X  "/1(X_idx)  "<X_idx>"
  signal_bus/1 -> get att_ff/1(signal_bus)

== system main_sim/claw_main/input processing/mode dependent stick processing/llh cmd ==
  mode : Inport  OutDataType=sfix(16)  OutScaling=2^0
  command_in : Inport  Port=2  OutDataType=sfix(16)  OutScaling=2^0
  signal_bus : Inport  Port=3  OutDataType=sfix(16)  OutScaling=2^0
  Assignment : Assignment  IndexOptions=Index vector (dialog)  Indices=[1 2 4]  OutputSizes=[1 1]
  Bus Selector : BusSelector  OutputSignals=mode_sw.llh_input_sw,y_meas.vehicle_origin
  Compare To Constant1 : simulink/Logic and Bit Operations/Compare To Constant  SystemSampleTime=-1  relop===  const=modes.pos  LogicOutDataTypeMode=boolean  ZeroCross=off
  LLh2NEh : utility_lib/LLh2NEh  SystemSampleTime=-1
  Logical Operator4 : Logic  AllPortsSameDT=off
  Multiport Switch2 : MultiPortSwitch  Inputs=2  zeroidx=on  SaturateOnIntegerOverflow=on
  Selector1 : Selector  InputPortWidth=4  IndexOptions=Index vector (dialog)  Indices=[1 2 4]  OutputSizes=1
  command_out : Outport  OutDataType=sfix(16)  OutScaling=2^0
  wires:
  Bus Selector/2 -> LLh2NEh/2  "<vehicle_origin>"
  command_in/1 -> Multiport Switch2/2, Assignment/1, Selector1/1
  Selector1/1 -> LLh2NEh/1
  LLh2NEh/1 -> Assignment/2
  Assignment/1 -> Multiport Switch2/3
  Multiport Switch2/1 -> command_out/1
  signal_bus/1 -> Bus Selector/1
  Compare To Constant1/1 -> Logical Operator4/1
  Bus Selector/1 -> Logical Operator4/2  "<llh_input_sw>"
  Logical Operator4/1 -> Multiport Switch2/1
  mode/1 -> Compare To Constant1/1

== system main_sim/claw_main/input processing/mode dependent stick processing/rampin vel_cmd ==
  mode : Inport  OutDataType=sfix(16)  OutScaling=2^0
  command_in : Inport  Port=2  OutDataType=sfix(16)  OutScaling=2^0
  NEh_dot : Inport  Port=3  OutDataType=sfix(16)  OutScaling=2^0
  Compare To Constant : simulink/Logic and Bit Operations/Compare To Constant  SystemSampleTime=-1  relop=<=  const=modes.att  LogicOutDataTypeMode=boolean  ZeroCross=off
  Compare To Constant1 : simulink/Logic and Bit Operations/Compare To Constant  SystemSampleTime=-1  relop===  const=modes.vel  LogicOutDataTypeMode=boolean  ZeroCross=off
  Constant : Constant  Value=MACH.dt/max(vel_cmd_ramp_time,MACH.dt)  OutDataType=sfix(16)  OutScaling=2^0
  Constant1 : Constant  OutDataType=sfix(16)  OutScaling=2^0
  Constant2 : Constant  Value=0  OutDataType=sfix(16)  OutScaling=2^0
  Logical Operator : Logic  AllPortsSameDT=off
  MinMax : MinMax  Function=max  Inputs=2  OutDataType=sfix(16)  OutScaling=2^0
  Product : Product  OutDataType=sfix(16)  OutScaling=2^0  RndMeth=Zero
  Product1 : Product  OutDataType=sfix(16)  OutScaling=2^0  RndMeth=Zero
  Sum : Sum  Inputs=-+|  OutDataType=sfix(16)  OutScaling=2^0
  Sum2 : Sum  Inputs=|++  OutDataType=sfix(16)  OutScaling=2^0
  Sum3 : Sum  Inputs=|+-  OutDataType=sfix(16)  OutScaling=2^0
  Switch : Switch  Threshold=0.5
  Switch1 : Switch  Threshold=0.5
  Unit Delay : UnitDelay  Orientation=left  SampleTime=-1
  Unit Delay1 : UnitDelay  SampleTime=-1
  Unit Delay2 : UnitDelay  Orientation=left  SampleTime=-1
  set vel cmd : Assignment  IndexOptions=Index vector (dialog)  Indices=[1 2 4]  OutputSizes=[1 1]
  vel cmd : Selector  InputPortWidth=4  IndexOptions=Index vector (dialog)  Indices=[1 2 4]  OutputSizes=1
  command_out : Outport  OutDataType=sfix(16)  OutScaling=2^0
  wires:
  Unit Delay2/1 -> Product1/2
  Logical Operator/1 -> Switch/2, Switch1/2
  Compare To Constant1/1 -> Logical Operator/2, Product1/1
  Compare To Constant/1 -> Logical Operator/1
  Unit Delay1/1 -> Compare To Constant/1
  mode/1 -> Unit Delay1/1, Compare To Constant1/1
  Unit Delay/1 -> Switch/3
  Switch/1 -> Unit Delay/1, Product/1
  NEh_dot/1 -> Sum/2
  Sum/1 -> Switch/1
  set vel cmd/1 -> command_out/1
  vel cmd/1 -> Sum2/1, Sum/1
  command_in/1 -> set vel cmd/1, vel cmd/1
  Sum2/1 -> set vel cmd/2
  Product1/1 -> Switch1/3
  Constant1/1 -> Switch1/1
  Switch1/1 -> Sum3/1
  Product/1 -> Sum2/2
  Sum3/1 -> MinMax/2
  Constant/1 -> Sum3/2
  MinMax/1 -> Product/2, Unit Delay2/1
  Constant2/1 -> MinMax/1

== system main_sim/claw_main/input processing/mode dependent stick processing/set command selection switches ==
  accel_cmd_sw : Inport  OutDataType=sfix(16)  OutScaling=2^0
  CLAW_mode : Inport  Port=2  OutDataType=sfix(16)  OutScaling=2^0
  Bus Creator : BusCreator
  Constant : Constant  Value=MACH.select_cmd_array  OutDataType=sfix(16)  OutScaling=2^0
  Demux : Demux  Outputs=[4 5 4 4]
  Reshape : Reshape
  Selector : Selector  NumberOfDimensions=2  IndexMode=Zero-based  InputPortWidth=3  IndexOptions=Select all,Index vector (port)  Indices=-1,1  OutputSizes=1
  modify for accel cmd submode : Subsystem
  select_cmd : Outport  OutDataType=sfix(16)  OutScaling=2^0
  wires:
  Constant/1 -> Selector/1
  CLAW_mode/1 -> Selector/2
  Selector/1 -> Reshape/1
  Demux/1 -> Bus Creator/1  "rate"
  Demux/2 -> Bus Creator/2  "att"
  Demux/3 -> Bus Creator/3  "vel"
  Demux/4 -> Bus Creator/4  "pos"
  Reshape/1 -> Demux/1
  modify for accel cmd submode/1(select_cmd) -> select_cmd/1
  Bus Creator/1 -> modify for accel cmd submode/1(select_cmd_in)
  accel_cmd_sw/1 -> modify for accel cmd submode/2(accel_cmd_sw)

== system main_sim/claw_main/input processing/mode dependent stick processing/table iv computation ==
  x_est : Inport  OutDataType=sfix(16)  OutScaling=2^0
  Bus Creator : BusCreator  Inputs=5
  Compare To Constant : simulink/Logic and Bit Operations/Compare To Constant  SystemSampleTime=-1  relop=>=  const=eow_boundary  LogicOutDataTypeMode=boolean  ZeroCross=off
  Constant : Constant  Value=2*constants.g  OutDataType=sfix(16)  OutScaling=2^0
  Constant1 : Constant  Value=sinA  OutDataType=sfix(16)  OutScaling=2^0
  Constant2 : Constant  Value=cosA  OutDataType=sfix(16)  OutScaling=2^0
  Constant3 : Constant  Value=N_rwy  OutDataType=sfix(16)  OutScaling=2^0
  Constant4 : Constant  Value=E_rwy  OutDataType=sfix(16)  OutScaling=2^0
  Dot Product : simulink/Math Operations/Dot Product  InputSameDT=on  OutDataType=sfix(16)  OutScaling=2^-10  DoSatur=off
  PreLookup Index Search : simulink_need_slupdate/PreLookup Index Search  bpData=tbl_eow  searchMode=Binary Search  cacheBpFlag=off  outputFlag=off  IndexDataType=uint32  extrapMode=Linear Extrapolation  rangeErrorMode=None
  PreLookup Index Search1 : simulink_need_slupdate/PreLookup Index Search  bpData=tbl_X  searchMode=Binary Search  cacheBpFlag=off  outputFlag=off  IndexDataType=uint32  extrapMode=Clip to Range  rangeErrorMode=None
  Product1 : Product  OutDataType=sfix(16)  OutScaling=2^0  RndMeth=Zero
  Product2 : Product  Inputs=*/  OutDataType=sfix(16)  OutScaling=2^0  RndMeth=Zero
  Product3 : Product  OutDataType=sfix(16)  OutScaling=2^0  RndMeth=Zero
  Sum1 : Sum  Inputs=|++  OutDataType=sfix(16)  OutScaling=2^0
  Sum2 : Sum  Inputs=-+|  OutDataType=sfix(16)  OutScaling=2^0
  Sum3 : Sum  Inputs=+|+  OutDataType=sfix(16)  OutScaling=2^0
  Sum4 : Sum  Inputs=|+-  OutDataType=sfix(16)  OutScaling=2^0
  get E : Selector  InputPortWidth=13  IndexOptions=Index vector (dialog)  Indices=8  OutputSizes=1
  get N : Selector  InputPortWidth=13  IndexOptions=Index vector (dialog)  Indices=7  OutputSizes=1
  get h : Selector  InputPortWidth=13  IndexOptions=Index vector (dialog)  Indices=9  OutputSizes=1
  get uvw : Selector  InputPortWidth=13  IndexOptions=Index vector (dialog)  Indices=4:6  OutputSizes=1
  table_bus : Outport  OutDataType=sfix(16)  OutScaling=2^0
  wires:
  get uvw/1 -> Dot Product/1, Dot Product/2
  get h/1 -> Sum1/1
  Constant/1 -> Product2/2
  Dot Product/1 -> Product2/1
  Product2/1 -> Sum1/2
  x_est/1 -> get h/1, get uvw/1, get N/1, get E/1
  Sum1/1 -> PreLookup Index Search/1, Compare To Constant/1, Bus Creator/2  "eow"
  PreLookup Index Search/1 -> Bus Creator/3  "eow_idx"
  get N/1 -> Sum2/2
  Sum2/1 -> Product3/1
  Product3/1 -> Sum3/1
  Constant2/1 -> Product3/2
  get E/1 -> Sum4/1
  Product1/1 -> Sum3/2
  Constant1/1 -> Product1/1
  Constant3/1 -> Sum2/1
  Constant4/1 -> Sum4/2
  Sum4/1 -> Product1/2
  Sum3/1 -> PreLookup Index Search1/1, Bus Creator/4  "X"
  Bus Creator/1 -> table_bus/1
  PreLookup Index Search1/1 -> Bus Creator/5  "X_idx"
  Compare To Constant/1 -> Bus Creator/1  "eow_large"

== system main_sim/claw_main/input processing/mode dependent stick processing/use table lookup pos cmds ==
  mode : Inport  OutDataType=sfix(16)  OutScaling=2^0
  command_in : Inport  Port=2  OutDataType=sfix(16)  OutScaling=2^0
  table_bus : Inport  Port=3  OutDataType=sfix(16)  OutScaling=2^0
  Assertion : Assertion  Enabled=off  AssertionFailFcn=assertioncb  StopWhenAssertionFail=off
  Bus Selector : BusSelector  OutputSignals=eow_idx,eow_large,X_idx,X
  Compare To Constant1 : simulink/Logic and Bit Operations/Compare To Constant  SystemSampleTime=-1  relop===  const=modes.pos  LogicOutDataTypeMode=boolean  ZeroCross=off
  Constant4 : Constant  Value=use_eow_as_iv  OutDataType=sfix(16)  OutScaling=2^0
  Logical Operator : Logic  AllPortsSameDT=off
  Relational Operator : RelationalOperator  LogicOutDataTypeMode=boolean  OutDataTypeStr=boolean
  Switch1 : Switch  Threshold=0.5
  Switch2 : Switch  Threshold=0.5
  Unit Delay : UnitDelay  SampleTime=-1
  pos cmd : Selector  InputPortWidth=4  IndexOptions=Index vector (dialog)  Indices=[1 2 4]  OutputSizes=1
  set pos cmd : Assignment  IndexOptions=Index vector (dialog)  Indices=[1 2 4]  OutputSizes=[1 1]
  use E/W to get pos cmds : Subsystem
  use X to get pos cmds : Subsystem
  command_out : Outport  OutDataType=sfix(16)  OutScaling=2^0
  wires:
  Logical Operator/1 -> Switch2/2, Unit Delay/1, Relational Operator/2
  Compare To Constant1/1 -> Logical Operator/2
  Constant4/1 -> Logical Operator/1
  mode/1 -> Compare To Constant1/1
  set pos cmd/1 -> command_out/1
  pos cmd/1 -> Switch2/3
  command_in/1 -> set pos cmd/1, pos cmd/1
  Switch2/1 -> set pos cmd/2
  use E/W to get pos cmds/1(pos_cmd_eow) -> Switch1/1
  use X to get pos cmds/1(pos_cmd_X) -> Switch1/3
  Switch1/1 -> Switch2/1
  Bus Selector/2 -> Switch1/2  "<eow_large>"
  table_bus/1 -> Bus Selector/1
  Bus Selector/1 -> use E/W to get pos cmds/1(eow_idx)  "<eow_idx>"
  Bus Selector/3 -> use X to get pos cmds/1(X_idx)  "<X_idx>"
  Bus Selector/4 -> use X to get pos cmds/2(X)  "<X>"
  Unit Delay/1 -> Relational Operator/1
  Relational Operator/1 -> Assertion/1

== system main_sim/claw_main/input processing/modify limits and apply to direct commands/apply surface locking ==
  u_meas : Inport  OutDataType=sfix(16)  OutScaling=2^0
  full_surf_in : Inport  Port=2  OutDataType=sfix(16)  OutScaling=2^0
  Bus Assignment : BusAssignment  AssignedSignals=full_surf_ulim,full_surf_llim
  Bus Selector : BusSelector  OutputSignals=full_surf_ulim,full_surf_cmd,full_surf_lock,full_surf_llim
  Multiport Switch : MultiPortSwitch  zeroidx=on
  Multiport Switch1 : MultiPortSwitch  zeroidx=on
  full_surf : Outport  OutDataType=sfix(16)  OutScaling=2^0
  wires:
  full_surf_in/1 -> Bus Selector/1, Bus Assignment/1
  Multiport Switch/1 -> Bus Assignment/2
  Multiport Switch1/1 -> Bus Assignment/3
  u_meas/1 -> Multiport Switch1/4, Multiport Switch/4
  Bus Assignment/1 -> full_surf/1
  Bus Selector/3 -> Multiport Switch1/1, Multiport Switch/1  "<full_surf_lock>"
  Bus Selector/1 -> Multiport Switch/2  "<full_surf_ulim>"
  Bus Selector/2 -> Multiport Switch/3, Multiport Switch1/3  "<full_surf_cmd>"
  Bus Selector/4 -> Multiport Switch1/2  "<full_surf_llim>"

== system main_sim/claw_main/input processing/modify limits and apply to direct commands/throt out of fuel limits ==
  full_surf_in : Inport  OutDataType=sfix(16)  OutScaling=2^0
  Bus Assignment : BusAssignment  AssignedSignals=full_surf_ulim,full_surf_llim
  Bus Selector3 : BusSelector  OutputSignals=full_surf_ulim,full_surf_llim
  throt out of fuel limits : model_lib/throt out of fuel limits  SystemSampleTime=-1
  full_surf : Outport  OutDataType=sfix(16)  OutScaling=2^0
  wires:
  Bus Selector3/1 -> throt out of fuel limits/1  "<full_surf_ulim>"
  Bus Selector3/2 -> throt out of fuel limits/2  "<full_surf_llim>"
  full_surf_in/1 -> Bus Selector3/1, Bus Assignment/1
  Bus Assignment/1 -> full_surf/1
  throt out of fuel limits/1 -> Bus Assignment/2
  throt out of fuel limits/2 -> Bus Assignment/3

== system main_sim/claw_main/input processing/select att_type/add tiebreaker for current att_type ==
  att_type_selected : Inport  OutDataType=sfix(16)  OutScaling=2^0
  priority_in : Inport  Port=2  OutDataType=sfix(16)  OutScaling=2^0
  Assignment1 : Assignment  IndexMode=Zero-based  IndexOptions=Index vector (port)  Indices=1  OutputSizes=length(att_type_numbers)+1
  Constant1 : Constant  Value=0.5  OutDataType=sfix(16)  OutScaling=2^0
  Selector : Selector  IndexMode=Zero-based  InputPortWidth=length(att_type_numbers)+1  IndexOptions=Index vector (port)  Indices=[1 3]  OutputSizes=1
  Sum1 : Sum  Inputs=|++  OutDataType=sfix(16)  OutScaling=2^0
  Unit Delay : UnitDelay  SampleTime=-1
  priority_out : Outport  OutDataType=sfix(16)  OutScaling=2^0
  wires:
  att_type_selected/1 -> Unit Delay/1
  priority_in/1 -> Selector/1, Assignment1/1
  Selector/1 -> Sum1/1
  Constant1/1 -> Sum1/2
  Sum1/1 -> Assignment1/2
  Unit Delay/1 -> Selector/2, Assignment1/3
  Assignment1/1 -> priority_out/1

== system main_sim/claw_main/input processing/select att_type/compute precond vars ==
  signal_bus : Inport  OutDataType=sfix(16)  OutScaling=2^0
  scoped_bus : Inport  Port=2  OutDataType=sfix(16)  OutScaling=2^0
  -sin_b : Selector  InputPortWidth=9  IndexOptions=Index vector (dialog)  Indices=1  OutputSizes=1
  -sin_theta : Selector  InputPortWidth=9  IndexOptions=Index vector (dialog)  Indices=7  OutputSizes=1
  Bus Creator : BusCreator  Inputs=6
  Bus Selector2 : BusSelector  OutputSignals=aero_env_est.qbar,aero_env_est.vel,aero_env_est.beta,y_meas.dircos
  Bus Selector4 : BusSelector  OutputSignals=dc_L2W
  Saturation : Saturate  UpperLimit=1  LowerLimit=-1
  Saturation1 : Saturate  UpperLimit=1  LowerLimit=-1
  Trigonometric Function : Trigonometry  Operator=cos
  abs_cos_b : Fcn  Expr=sqrt(1-u(1)^2)
  abs_cos_beta : Abs
  abs_cos_gamma_rw : Abs
  abs_cos_theta : Fcn  Expr=sqrt(1-u(1)^2)
  abs_vel_rw : Abs
  cos_gamma_rw : Selector  InputPortWidth=9  IndexOptions=Index vector (dialog)  Indices=9  OutputSizes=1
  precond_vars : Outport  OutDataType=sfix(16)  OutScaling=2^0
  wires:
  Bus Selector4/1 -> cos_gamma_rw/1  "<dc_L2W>"
  Bus Selector2/1 -> Bus Creator/1  "<qbar>"
  Bus Selector2/2 -> abs_vel_rw/1  "<vel>"
  Bus Selector2/3 -> Trigonometric Function/1  "<beta>"
  Bus Selector2/4 -> -sin_theta/1, -sin_b/1  "<dircos>"
  Trigonometric Function/1 -> abs_cos_beta/1
  -sin_b/1 -> Saturation1/1
  -sin_theta/1 -> Saturation/1
  cos_gamma_rw/1 -> abs_cos_gamma_rw/1
  abs_vel_rw/1 -> Bus Creator/2  "abs_vel_rw"
  abs_cos_beta/1 -> Bus Creator/3  "abs_cos_beta"
  abs_cos_theta/1 -> Bus Creator/4  "abs_cos_theta"
  abs_cos_b/1 -> Bus Creator/5  "abs_cos_b"
  abs_cos_gamma_rw/1 -> Bus Creator/6  "abs_cos_gamma_rw"
  Saturation/1 -> abs_cos_theta/1
  Saturation1/1 -> abs_cos_b/1
  signal_bus/1 -> Bus Selector2/1
  Bus Creator/1 -> precond_vars/1
  scoped_bus/1 -> Bus Selector4/1

== system main_sim/claw_main/input processing/select att_type/evaluate preconditions ==
  precond_vars : Inport  OutDataType=sfix(16)  OutScaling=2^0
  Bus Selector5 : BusSelector  OutputSignals=abs_cos_b,abs_cos_theta,abs_vel_rw,abs_cos_beta,abs_cos_gamma_rw,qbar
  Compare To Constant : simulink/Logic and Bit Operations/Compare To Constant  SystemSampleTime=-1  relop=>=  const=1  LogicOutDataTypeMode=boolean  ZeroCross=off
  Compare To Constant1 : simulink/Logic and Bit Operations/Compare To Constant  SystemSampleTime=-1  relop=>=  const=cos(pi/3)  LogicOutDataTypeMode=boolean  ZeroCross=off
  Compare To Constant2 : simulink/Logic and Bit Operations/Compare To Constant  SystemSampleTime=-1  relop=>=  const=0.1  LogicOutDataTypeMode=boolean  ZeroCross=off
  Compare To Constant3 : simulink/Logic and Bit Operations/Compare To Constant  SystemSampleTime=-1  relop=>=  const=cos(pi/3)  LogicOutDataTypeMode=boolean  ZeroCross=off
  Compare To Constant4 : simulink/Logic and Bit Operations/Compare To Constant  SystemSampleTime=-1  relop=>=  const=cos(pi/3)  LogicOutDataTypeMode=boolean  ZeroCross=off
  Compare To Constant5 : simulink/Logic and Bit Operations/Compare To Constant  SystemSampleTime=-1  relop=>=  const=1  LogicOutDataTypeMode=boolean  ZeroCross=off
  Constant : Constant  Value=boolean(0)  OutDataType=sfix(16)  OutScaling=2^0
  Logical Operator : Logic  Inputs=4  AllPortsSameDT=off  OutDataTypeMode=boolean  OutDataTypeStr=boolean
  Mux : Mux  Inputs=6
  precond_satisfied : Outport  OutDataType=sfix(16)  OutScaling=2^0
  wires:
  Compare To Constant/1 -> Logical Operator/1
  Compare To Constant1/1 -> Logical Operator/2
  Compare To Constant2/1 -> Logical Operator/3
  Compare To Constant3/1 -> Mux/3, Mux/4
  Compare To Constant4/1 -> Mux/2
  Bus Selector5/1 -> Compare To Constant4/1  "<abs_cos_b>"
  Bus Selector5/2 -> Compare To Constant3/1  "<abs_cos_theta>"
  Bus Selector5/3 -> Compare To Constant/1  "<abs_vel_rw>"
  Bus Selector5/4 -> Compare To Constant1/1  "<abs_cos_beta>"
  Bus Selector5/5 -> Compare To Constant2/1  "<abs_cos_gamma_rw>"
  Logical Operator/1 -> Mux/5, Mux/6
  Constant/1 -> Mux/1
  Compare To Constant5/1 -> Logical Operator/4
  Bus Selector5/6 -> Compare To Constant5/1  "<qbar>"
  precond_vars/1 -> Bus Selector5/1
  Mux/1 -> precond_satisfied/1

== system main_sim/claw_main/input processing/select att_type/select best att_type ==
  vec : Inport  OutDataType=sfix(16)  OutScaling=2^0
  Constant4 : Constant  Value=0:length(att_type_numbers)  OutDataType=sfix(16)  OutScaling=2^0
  Constant5 : Constant  Value=length(att_type_numbers)  OutDataType=sfix(16)  OutScaling=2^0
  MinMax3 : MinMax  Function=max  OutDataType=sfix(16)  OutScaling=2^0  SaturateOnIntegerOverflow=on  InputSameDT=on
  MinMax4 : MinMax  OutDataType=sfix(16)  OutScaling=2^0  SaturateOnIntegerOverflow=on  InputSameDT=on
  Sum2 : Sum  Inputs=+-|  OutDataType=sfix(16)  OutScaling=2^0  SaturateOnIntegerOverflow=on
  argmax1 : Switch  Threshold=-eps  SaturateOnIntegerOverflow=on
  idx_max : Outport  OutDataType=sfix(16)  OutScaling=2^0
  wires:
  vec/1 -> MinMax3/1, Sum2/1
  Sum2/1 -> argmax1/2
  Constant4/1 -> argmax1/1
  Constant5/1 -> argmax1/3
  argmax1/1 -> MinMax4/1
  MinMax3/1 -> Sum2/2
  MinMax4/1 -> idx_max/1
